simulink model "halfCarVerif"  (R2017b)
settings: Solver=VariableStepAuto  StartTime=0.0  StopTime=10.0  RelTol=1e-3
settings Model: Creator=cs756  LastModifiedBy=cs756

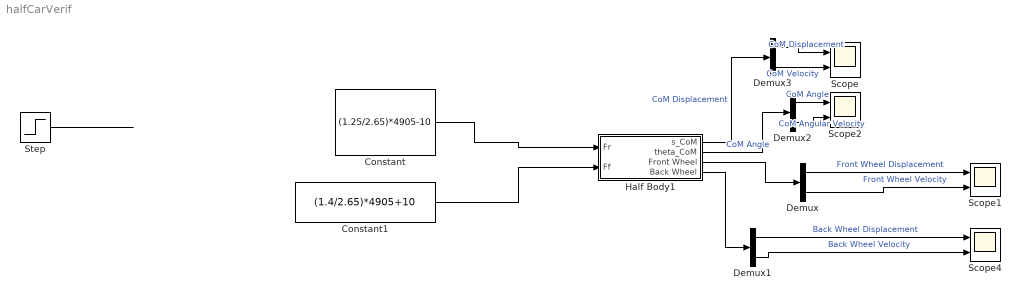
== system halfCarVerif ==
  Constant : Constant  Value=(1.25/2.65)*4905-10
  Constant1 : Constant  Value=(1.4/2.65)*4905+10
  Demux{,1..3} (4 alike) : Demux  Outputs=2
  Half Body1 : Subsystem  mask{g=9.81, I=600, mb=500, a=1.25, b=1.4}
      mask prompts: I "Moment of Inertia"; mb "Body Mass"
  Scope{,1..2,4} (4 alike) : Scope  NumInputPorts=2
  Step : Step  SampleTime=0
  wires:
  Step/1 -> ?
  Half Body1/1(s_CoM) -> Demux3/1  "CoM Displacement"
  Half Body1/3(Front Wheel) -> Demux/1
  Half Body1/4(Back Wheel) -> Demux1/1
  Constant/1 -> Half Body1/1(Fr)
  Constant1/1 -> Half Body1/2(Ff)
  Half Body1/2(theta_CoM) -> Demux2/1  "CoM Angle"
  Demux/2 -> Scope1/2  "Front Wheel Velocity"
  Demux/1 -> Scope1/1  "Front Wheel Displacement"
  Demux1/1 -> Scope4/1  "Back Wheel Displacement"
  Demux1/2 -> Scope4/2  "Back Wheel Velocity"
  Demux3/1 -> Scope/1  "CoM Displacement"
  Demux3/2 -> Scope/2  "CoM Velocity"
  Demux2/1 -> Scope2/1  "CoM Angle"
  Demux2/2 -> Scope2/2  "CoM Angular Velocity"

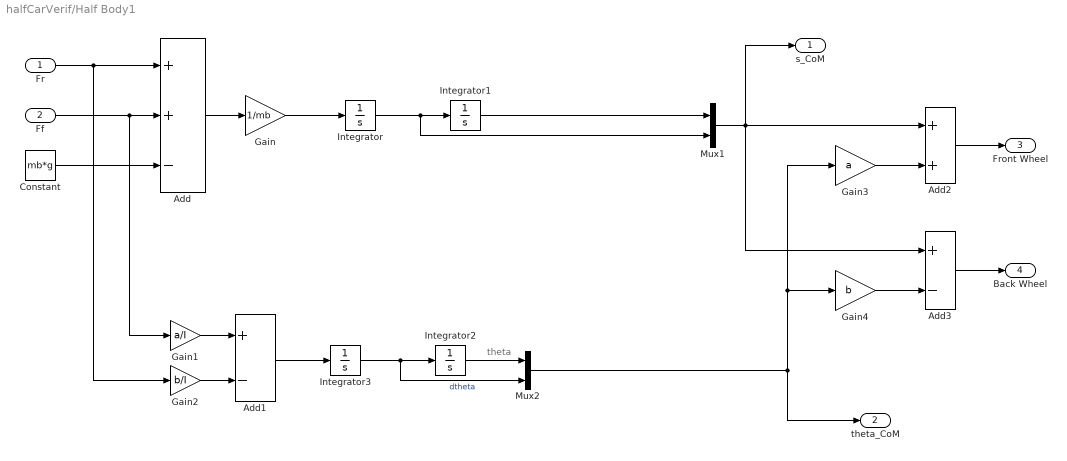
== system halfCarVerif/Half Body1 ==
  note: theta
  Fr : Inport
  Ff : Inport  Port=2
  Add : Sum  Inputs=++-
  Add1 : Sum  Inputs=+-
  Add2 : Sum
  Add3 : Sum  Inputs=+-
  Constant : Constant  Value=mb*g
  Gain : Gain  Gain=1/mb
  Gain1 : Gain  Gain=a/I
  Gain2 : Gain  Gain=b/I
  Gain3 : Gain  Gain=a
  Gain4 : Gain  Gain=b
  Integrator{,1..3} (4 alike) : Integrator
  Mux1 : Mux  Inputs=2
  Mux2 : Mux  Inputs=2
  s_CoM : Outport
  theta_CoM : Outport  Port=2
  Front Wheel : Outport  Port=3
  Back Wheel : Outport  Port=4
  wires:
  Fr/1 -> Gain2/1, Add/1
  Constant/1 -> Add/3
  Add/1 -> Gain/1
  Gain/1 -> Integrator/1
  Integrator/1 -> Mux1/2, Integrator1/1
  Ff/1 -> Gain1/1, Add/2
  Gain2/1 -> Add1/2
  Gain1/1 -> Add1/1
  Integrator3/1 -> Mux2/2, Integrator2/1  "dtheta"
  Add1/1 -> Integrator3/1
  Integrator1/1 -> Mux1/1
  Integrator2/1 -> Mux2/1
  Gain3/1 -> Add2/2
  Gain4/1 -> Add3/2
  Add2/1 -> Front Wheel/1
  Add3/1 -> Back Wheel/1
  Mux2/1 -> Gain3/1, Gain4/1, theta_CoM/1
  Mux1/1 -> s_CoM/1, Add2/1, Add3/1
